simulink model "CONTROL_diferencia_simulink"  (R2025a)
settings: Solver=FixedStepAuto  StartTime=0.0  StopTime=inf  FixedStep=0.001  RelTol=1e-3
undefined symbols (not defined in the file): Standard_Devices, UDP_Protocol
libraries: sldrtlib x1
settings Model: Creator=Mathias Voigt  LastModifiedBy=adria
settings SolverCC: AlgebraicLoopSolver=TrustRegion
settings DebuggingCC: UnconnectedInputMsg=warning  UnconnectedOutputMsg=warning  UnconnectedLineMsg=warning
settings ModelReferenceCC: EnableRefExpFcnMdlSchedulingChecks=on
settings SFSimCC: CustomCodeUndefinedFunction=UseInterfaceOnly
settings RTWCC: GPUComputeCapability=3.5

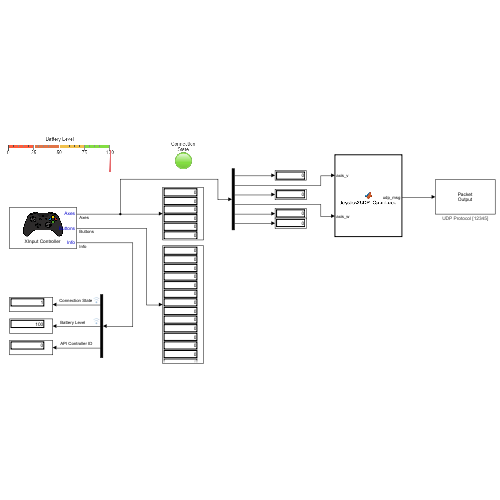
[thumbnail: Simulink's stored preview of the top-level diagram]
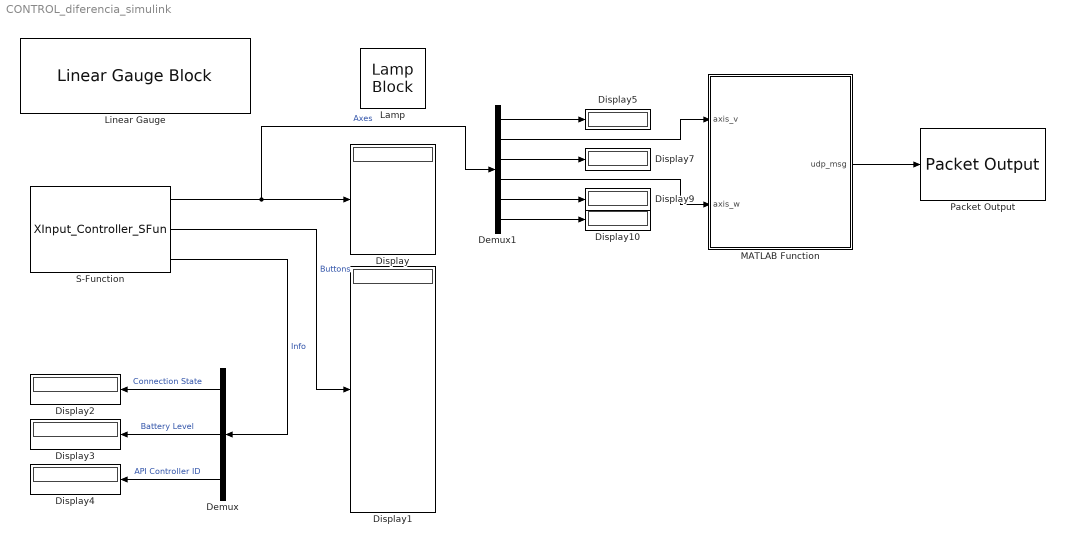
== system CONTROL_diferencia_simulink ==
  Demux : Demux  Outputs=3
  Demux1 : Demux  Outputs=6
  Display{,1..5,7,9..10} (9 alike) : Display
  Lamp : LampBlock  DefaultColor=[192.0, 192.0, 192.0]
  Linear Gauge : LinearGaugeBlock  TickInterval=25  FontColor=[0.0, 0.0, 0.0]
  MATLAB Function : MATLAB Function  TreatAsAtomicUnit=on
  Packet Output : sldrtlib/Packet Output  SampleTime=0.1  MaxMissedTicks=10  ShowMissedTicks=off  YieldWhenWaiting=off  DrvName=Standard_Devices/UDP_Protocol  DrvAddress=12345  DrvOptions=[0 12345 49 57 50 46 49 54 56 46 49 51 55 46 52 55 0 0 0 0 0 0 0 0 0 0 0 0 0 0 0 0 0 0 0 0 0 0 0 0 0 0 0 0 0 0 0 0 0 0 0 0 0 0 0 0 0 0 0 0 0 0 0 0 0 0 0 0 0 0 0 0 0 0 0 0 0 0 0 0 0 0 0 0 0 0 0 0 0 0 0 0 0 0 0 0 0 0 0 0 0 0 0 0 0 0 0 0 0 0 0 0 0 0 0 0 0 0 0 0 0 0 0 0 0 0 0 0 0 0 0 0 0 0 0 0 0 0 0 0 0 0 0 0 0 0 0 0 0 0 0 0 0 0 0 0 0 0 0 0 0 0 0 0 0 0 0 0 0 0 0 0 0 0 0 0 0 0 0 0 0 0 0 0 0 0 0 0 0 0 0 0 0 0 0 0 0 0 0 0 0 0 0 0 0 0 0 0 0 0 0 0 0 0 0 0 0 0 0 0 0 0 0 0 0 0 0 0 0 0 0 0 0 0 0 0 0 0 0 0 0 0 0 0 0 0 0 0 0 0 0 0 0 0 0 0]  PacketSize=16  DataTypes='16*uint8'  ShowReady=off  ShowError=off  PacketID=1  ByteOrder=1  InitialValue=[]  FinalValue=[]
      settings: AttributesFormatString=UDP Protocol [12345]
  S-Function : S-Function  FunctionName=XInput_Controller_SFun  Parameters=ControllerID  SFunctionDeploymentMode=off  EnableBusSupport=off  mask(XInput Controller){ControllerID=1}
      mask help:
      | This Block will allow you to use XInput Controllers in Simulink.
      | XInput is the most Supported API.
      | Works with XBOX 360 and XBOX ONE Controllers.
      |
      | Use 'DEMUX' to access Signals
      | Output_1 [1x6]
      |   Analog Left X, Analog Left Y,
      |   Analog Right X, Analog Right Y,
      |   Left Trigger, Right Trigger
      | Output_2 [1x14]
      |   Up, Down, Left, Right,
      |   Start, Back, Left Stick, Right Stick,
      |   Left Shoulder, Right Shoulder,
      |   A, B, X, Y
      | Output_3 [1x3]
      |   Connection State, Battery Level (1-4), Controller ID
      mask init:
      | ControllerID;   
      | blk = gcb; 
      | get_String = get_param(blk,'ControllerID');
      | ControllerID = str2double(get_String);
      mask Help:
      | Based on Microsoft XInput API
      | Therefore the maximum of conneced Gamepads per PC is 4. First Gamepad has Controller ID 1.
      | 
      | Reference:
      | https://docs.microsoft.com/en-us/windows/win32/api/_xinput/
      | 
      | Tutorial:
      | https://docs.microsoft.com/en-us/windows/win32/xinput/getting-started-with-xinput
      | 
      | Info:
      | The Analog Sticks Deadzone is coded to:
      | Deadzone = 6144;
      | 0 <= Deadzone <= 65534
      | This is smaller then Microsoft default.
      | 
      | created by Mathias Voigt
      | Technische Universität Dresden
      | 2019
      mask TypeOptions ControllerID: 1 | 2 | 3 | 4
      mask DialogControl ParameterGroupVar Prompt: Controller ID
      mask Display:
      | %% Set Block picture from user Data
      | %  (permanent, picture file not needed)
      | %  see persistent_image_allocation.m
      | 
      | %get the picture data
      | UserDataStrut = get_param(gcb, 'UserData');
      | image(UserDataStrut.Image, [0.2, 0.3, 0.6, 0.6])
      | 
      | 
      | 
      | % conventional method (does not save picture data in Simulink)
      | % image('XBOX_One_Controller_Icon.png', [0.2, 0.3, 0.6, 0.6])
      | 
      | %% Create Port Labels
      | color('blue');
      | port_label('output', 1, 'Axes');
      | port_label('output', 2, 'Buttons');
      | port_label('output', 3, 'Info');
      | 
      | 
      | %% Create S-Function Block Name
      | color('black');
      | text(0.5, 0.1, 'XInput Controller',...
      |      'horizontalAlignment', 'center',...
      |      'verticalAlignment', 'bottom');
  wires:
  S-Function/2 -> Display1/1  "Buttons"
  S-Function/1 -> Demux1/1, Display/1  "Axes"
  Demux/1 -> Display2/1  "Connection State"
  Demux/2 -> Display3/1  "Battery Level"
  Demux/3 -> Display4/1  "API Controller ID"
  S-Function/3 -> Demux/1  "Info"
  Demux1/1 -> Display5/1
  Demux1/2 -> MATLAB Function/1(axis_v)
  Demux1/3 -> Display7/1
  Demux1/4 -> MATLAB Function/2(axis_w)
  Demux1/5 -> Display9/1
  Demux1/6 -> Display10/1
  MATLAB Function/1(udp_msg) -> Packet Output/1

== matlab function CONTROL_diferencia_simulink/MATLAB Function ==
  data: axis_v input; udp_msg output; axis_w input
function udp_msg = Joystick2UDP_OpenLoop(axis_v, axis_w)
%#codegen
% Mensaje ASCII compatible con ESP32

%% Cinemática (igual que antes)
R = 0.05;
L = 0.20;

v = axis_v * 0.8;
w = axis_w * 4.0;

omega_r = (2*v + w*L) / (2*R);
omega_l = (2*v - w*L) / (2*R);

omega_max = 10;
vel_r = (omega_r / omega_max) * 100;
vel_l = (omega_l / omega_max) * 100;

vel_r = min(max(vel_r, -100), 100);
vel_l = min(max(vel_l, -100), 100);

%% STRING ASCII
msg = sprintf('%.1f,%.1f', vel_l, vel_r);

%% BUFFER FIJO (Packet Output)
udp_msg = zeros(1,16,'uint8');   % 16 bytes fijos
msg_uint8 = uint8(msg);

udp_msg(1:length(msg_uint8)) = msg_uint8;
udp_msg(length(msg_uint8)+1) = 0;  % NULL TERMINATOR
end
